simulink model "pure_pursuit"  (R2024b)
settings: Solver=VariableStepAuto  StartTime=0.0  StopTime=10.0  FixedStep=T  RelTol=1e-3
settings Model: DataDictionary=wrapper2.sldd  Creator=maciej  LastModifiedBy=maciej

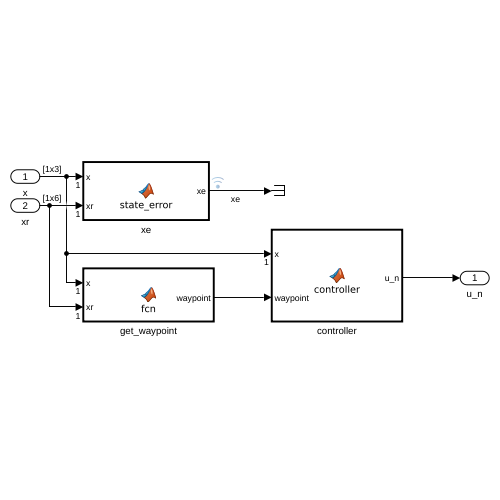
[thumbnail: Simulink's stored preview of the top-level diagram]
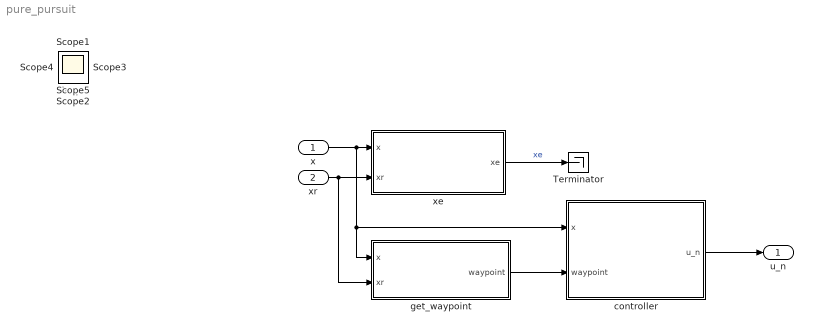
== system pure_pursuit ==
  x : Inport  PortDimensions=[1 3]
  xr : Inport  Port=2  PortDimensions=[1 6]
  Terminator : Terminator
  controller : MATLAB Function  TreatAsAtomicUnit=on
  get_waypoint : MATLAB Function  TreatAsAtomicUnit=on
  xe : MATLAB Function  TreatAsAtomicUnit=on
  u_n : Outport
  Scope{,1..5} (6 alike) : Scope
  wires:
  xr/1 -> get_waypoint/2(xr), xe/2(xr)
  get_waypoint/1(waypoint) -> controller/2(waypoint)
  xe/1(xe) -> Terminator/1  "xe"
  x/1 -> controller/1(x), get_waypoint/1(x), xe/1(x)
  controller/1(u_n) -> u_n/1

== matlab function pure_pursuit/get_waypoint ==
  data: x input; waypoint output; xr input
function waypoint = fcn(x, xr)
    waypoint = [x(1) + 50, xr(3)];
end

== matlab function pure_pursuit/xe ==
  data: x input; xe output; xr input
function xe = state_error(x, xr)
    c = cos(x(3));
    s = sin(x(3));
    dx = [xr(1) - x(1); xr(3) - x(2); xr(5) - x(3)];

    xe = [c s 0; -s c 0; 0 0 1] * dx;
end

== matlab function pure_pursuit/controller ==
  data: x input; u_n output; waypoint input
function u_n = controller(x, waypoint)
    persistent pp

    if isempty(pp)
        pp = controllerPurePursuit;
        pp.DesiredLinearVelocity = 1;
        pp.MaxAngularVelocity = 6;
    end

    pp.Waypoints = waypoint;
    [v, w] = pp(x);

    u_n = [v; w];
end
